simulink model "grid_loop"  (R2022b)
settings: Solver=VariableStepAuto  StartTime=0.0  StopTime=2  RelTol=1e-3
settings Model: Creator=stefanopanzieri  LastModifiedBy=stefanopanzieri

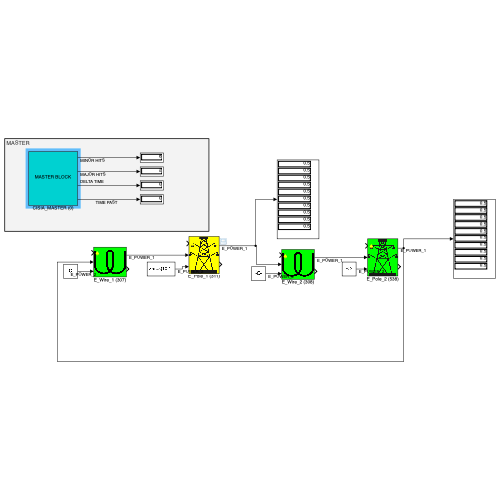
[thumbnail: Simulink's stored preview of the top-level diagram]
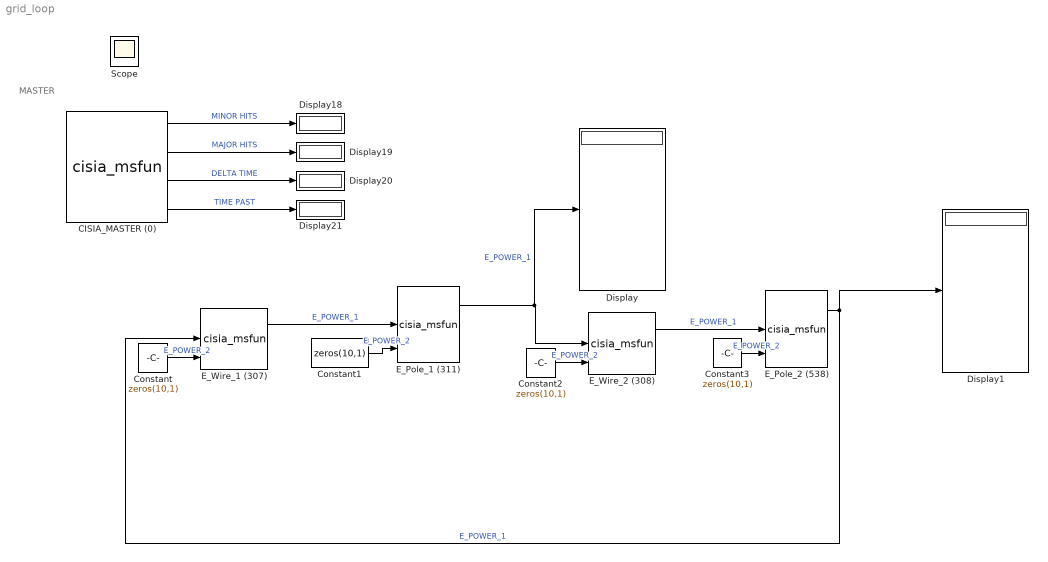
== system grid_loop ==
  note: MASTER
  CISIA_MASTER (0) : M-S-Function  FunctionName=cisia_msfun  Parameters=Parameter1, Parameter2, Parameter3, resources, Parameter4, Parameter5, Parameter6, Parameter7, Parameter8, Parameter9,Parameter11,Parameter12  mask(S-function:msfcn_unit_delay){Parameter1='CISIA_MASTER', Parameter2=[1], Parameter3='MicroGrid', resources=off, Parameter4=on, Parameter5=off, Parameter6=off, Parameter7=off, Parameter8=0.001, Parameter9=off, Parameter11=on, Parameter12=off}
      mask prompts: Parameter1 "entity name"; Parameter2 "sampling time"; Parameter3 "project"; resources "Save status at each major hit"; Parameter4 "Show Operative Levels with colors"; Parameter5 "Load Entities from file"; Parameter6 "Load Start from Mask"; Parameter7 "Real Time"; Parameter8 "Real Time Hit (sec)"; Parameter9 "Skip saving"; Parameter11 "Show unconnected"; Parameter12 "Save port values"
      mask help:
      | MASTER BLOCK
      | v.2.0
      mask Display: disp('MASTER BLOCK')
  Constant{,1..3} (4 alike) : Constant  Value=zeros(10,1)
  Display{,1,18..21} (6 alike) : Display
  E_Pole_1 (311) : M-S-Function  FunctionName=cisia_msfun  Parameters=Parameter1, Parameter2, Parameter3, resources, Parameter10, codeupdate, step_received, step_computed, dynamic_computed, step_sended, id_entity, id_project, id_type, name_type, color  mask(S-function:msfcn_unit_delay){Parameter1='E_Pole_1', Parameter2=1, Parameter3='', resources=|, Parameter10=off, codeupdate=off, step_received=|, step_computed=, dynamic_computed=, step_sended=|, id_entity=311, id_project=29, id_type=68, name_type=Electric_Pole, color=#FFFFFF}
      mask resources=|
      | *** INPUT RESOURCES ***
      | NUM_INPUTS 3
      | FLAME (1)
      | E_POWER_1 (10)
      | E_POWER_2 (10)
      |
      | *** STATE VARIABLES ***
      | NUM_VARIABLES 5
      | Operative_Level(NUMERIC)(1)(1)
      | Mechanical_Fault(NUMERIC)(1)(0.5)
      | Fire_Fault(NUMERIC)(1)(0)
      | Physical_Fault(NUMERIC)(1)(0)
      | Power_Gen(NUMERIC_ARRAY)(10)(0  0  0  0  0  0  0  0  0  0)
      |
      | *** OUTPUT RESOURCES ***
      | NUM_OUTPUTS 2
      | E_POWER_1 (10)
      | E_POWER_2 (10)
      mask step_received=|
      | Power_Gen=max(E_POWER_1,E_POWER_2);
      |
      | Fire_Fault=FLAME;
      |
      | Physical_Fault=max(Fire_Fault,Mechanical_Fault);
      |
      | Operative_Level=1-Physical_Fault;
      mask step_sended=|
      | E_POWER_1=min(Power_Gen,(1-Physical_Fault)*ones(size(Power_Gen)));
      |
      | E_POWER_2=min(Power_Gen,(1-Physical_Fault)*ones(size(Power_Gen)));
      mask prompts: Parameter1 "entity name"; Parameter2 "sampling time"; Parameter3 "project"; resources "input resources and state variables"; Parameter10 "Bring state variables to output"; codeupdate "update code from mask"
      mask help: This is a level-2 MATLAB file S-function which demonstrates CISIA entity
      mask DialogControl Container1 Prompt: All parameters
      mask Display: image('Icons/Electric_Pole.png');port_label('input',1,'\color{yellow}\spadesuit','texmode','on')
  E_Pole_2 (538) : M-S-Function  FunctionName=cisia_msfun  Parameters=Parameter1, Parameter2, Parameter3, resources, Parameter10, codeupdate, step_received, step_computed, dynamic_computed, step_sended, id_entity, id_project, id_type, name_type, color  mask(S-function:msfcn_unit_delay){Parameter1='E_Pole_2', Parameter2=1, Parameter3='', resources=|, Parameter10=off, codeupdate=off, step_received=|, step_computed=, dynamic_computed=, step_sended=|, id_entity=538, id_project=29, id_type=68, name_type=Electric_Pole, color=#FFFFFF}
      mask resources=|
      | *** INPUT RESOURCES ***
      | NUM_INPUTS 3
      | FLAME (1)
      | E_POWER_1 (10)
      | E_POWER_2 (10)
      |
      | *** STATE VARIABLES ***
      | NUM_VARIABLES 5
      | Operative_Level(NUMERIC)(1)(1)
      | Mechanical_Fault(NUMERIC)(1)(0)
      | Fire_Fault(NUMERIC)(1)(0)
      | Physical_Fault(NUMERIC)(1)(0)
      | Power_Gen(NUMERIC_ARRAY)(10)(0  0  0  0  0  0  0  0  0  0)
      |
      | *** OUTPUT RESOURCES ***
      | NUM_OUTPUTS 2
      | E_POWER_1 (10)
      | E_POWER_2 (10)
      mask step_received=|
      | Power_Gen=max(E_POWER_1,E_POWER_2);
      |
      | Fire_Fault=FLAME;
      |
      | Physical_Fault=max(Fire_Fault,Mechanical_Fault);
      |
      | Operative_Level=1-Physical_Fault;
      mask step_sended=|
      | E_POWER_1=min(Power_Gen,(1-Physical_Fault)*ones(size(Power_Gen)));
      |
      | E_POWER_2=min(Power_Gen,(1-Physical_Fault)*ones(size(Power_Gen)));
      mask prompts: Parameter1 "entity name"; Parameter2 "sampling time"; Parameter3 "project"; resources "input resources and state variables"; Parameter10 "Bring state variables to output"; codeupdate "update code from mask"
      mask help: This is a level-2 MATLAB file S-function which demonstrates CISIA entity
      mask DialogControl Container1 Prompt: All parameters
      mask Display: image('Icons/Electric_Pole.png');port_label('input',1,'\color{yellow}\spadesuit','texmode','on')
  E_Wire_1 (307) : M-S-Function  FunctionName=cisia_msfun  Parameters=Parameter1, Parameter2, Parameter3, resources, Parameter10, codeupdate, step_received, step_computed, dynamic_computed, step_sended, id_entity, id_project, id_type, name_type, color  mask(S-function:msfcn_unit_delay){Parameter1='E_Wire_1', Parameter2=1, Parameter3='', resources=|, Parameter10=off, codeupdate=off, step_received=|, step_computed=, dynamic_computed=, step_sended=|, id_entity=307, id_project=29, id_type=67, name_type=Electric_Wire, color=#FFFFFF}
      mask resources=|
      | *** INPUT RESOURCES ***
      | NUM_INPUTS 3
      | FLAME (1)
      | E_POWER_1 (10)
      | E_POWER_2 (10)
      |
      | *** STATE VARIABLES ***
      | NUM_VARIABLES 5
      | Operative_Level(NUMERIC)(1)(1)
      | Mechanical_Fault(NUMERIC)(1)(0)
      | Fire_Fault(NUMERIC)(1)(0)
      | Physical_Fault(NUMERIC)(1)(0)
      | Power_Gen(NUMERIC_ARRAY)(10)(0  0  0  0  0  0  0  0  0  0)
      |
      | *** OUTPUT RESOURCES ***
      | NUM_OUTPUTS 2
      | E_POWER_1 (10)
      | E_POWER_2 (10)
      mask step_received=|
      | Power_Gen=max(E_POWER_1,E_POWER_2);
      |
      | Fire_Fault=FLAME;
      |
      | Physical_Fault=max(Fire_Fault,Mechanical_Fault);
      |
      | Operative_Level=1-Physical_Fault;
      mask step_sended=|
      | E_POWER_1=min(Power_Gen,(1-Physical_Fault)*ones(size(Power_Gen)));
      |
      | E_POWER_2=min(Power_Gen,(1-Physical_Fault)*ones(size(Power_Gen)));
      mask prompts: Parameter1 "entity name"; Parameter2 "sampling time"; Parameter3 "project"; resources "input resources and state variables"; Parameter10 "Bring state variables to output"; codeupdate "update code from mask"
      mask help: This is a level-2 MATLAB file S-function which demonstrates CISIA entity
      mask DialogControl Container1 Prompt: All parameters
      mask Display: image('Icons/Electric_Wire.png');port_label('input',1,'\color{yellow}\spadesuit','texmode','on')
  E_Wire_2 (308) : M-S-Function  FunctionName=cisia_msfun  Parameters=Parameter1, Parameter2, Parameter3, resources, Parameter10, codeupdate, step_received, step_computed, dynamic_computed, step_sended, id_entity, id_project, id_type, name_type, color  mask(S-function:msfcn_unit_delay){Parameter1='E_Wire_2', Parameter2=1, Parameter3='', resources=|, Parameter10=off, codeupdate=off, step_received=|, step_computed=, dynamic_computed=, step_sended=|, id_entity=308, id_project=29, id_type=67, name_type=Electric_Wire, color=#FFFFFF}
      mask resources=|
      | *** INPUT RESOURCES ***
      | NUM_INPUTS 3
      | FLAME (1)
      | E_POWER_1 (10)
      | E_POWER_2 (10)
      |
      | *** STATE VARIABLES ***
      | NUM_VARIABLES 5
      | Operative_Level(NUMERIC)(1)(1)
      | Mechanical_Fault(NUMERIC)(1)(0)
      | Fire_Fault(NUMERIC)(1)(0)
      | Physical_Fault(NUMERIC)(1)(0)
      | Power_Gen(NUMERIC_ARRAY)(10)(0  0  0  0  0  0  0  0  0  0)
      |
      | *** OUTPUT RESOURCES ***
      | NUM_OUTPUTS 2
      | E_POWER_1 (10)
      | E_POWER_2 (10)
      mask step_received=|
      | Power_Gen=max(E_POWER_1,E_POWER_2);
      |
      | Fire_Fault=FLAME;
      |
      | Physical_Fault=max(Fire_Fault,Mechanical_Fault);
      |
      | Operative_Level=1-Physical_Fault;
      mask step_sended=|
      | E_POWER_1=min(Power_Gen,(1-Physical_Fault)*ones(size(Power_Gen)));
      |
      | E_POWER_2=min(Power_Gen,(1-Physical_Fault)*ones(size(Power_Gen)));
      mask prompts: Parameter1 "entity name"; Parameter2 "sampling time"; Parameter3 "project"; resources "input resources and state variables"; Parameter10 "Bring state variables to output"; codeupdate "update code from mask"
      mask help: This is a level-2 MATLAB file S-function which demonstrates CISIA entity
      mask DialogControl Container1 Prompt: All parameters
      mask Display: image('Icons/Electric_Wire.png');port_label('input',1,'\color{yellow}\spadesuit','texmode','on')
  Scope : Scope
  wires:
  CISIA_MASTER (0)/2 -> Display19/1  "MAJOR HITS"
  CISIA_MASTER (0)/1 -> Display18/1  "MINOR HITS"
  CISIA_MASTER (0)/4 -> Display21/1  "TIME PAST"
  CISIA_MASTER (0)/3 -> Display20/1  "DELTA TIME"
  E_Wire_1 (307)/1 -> E_Pole_1 (311)/2  "E_POWER_1"
  E_Pole_1 (311)/1 -> Display/1, E_Wire_2 (308)/2  "E_POWER_1"
  E_Wire_2 (308)/1 -> E_Pole_2 (538)/2  "E_POWER_1"
  E_Pole_2 (538)/1 -> Display1/1, E_Wire_1 (307)/2  "E_POWER_1"
  Constant/1 -> E_Wire_1 (307)/3  "E_POWER_2"
  Constant1/1 -> E_Pole_1 (311)/3  "E_POWER_2"
  Constant2/1 -> E_Wire_2 (308)/3  "E_POWER_2"
  Constant3/1 -> E_Pole_2 (538)/3  "E_POWER_2"
